simulink model "decision_stateflow"  (R2024b)
settings: Solver=ode1  StartTime=0.0  StopTime=10.0  FixedStep=0.01  RelTol=1e-3
undefined symbols (not defined in the file): U8Driver, U8DriverState, U8Ref_vel, U8RSPA, U8RSPAState
settings Model: ParamWorkspaceSource=ReferencedWorkspace  Creator=USER  LastModifiedBy=USER
settings OptimizationCC: DefaultParameterBehavior=Inlined  OptimizeBlockIOStorage=off  BufferReuse=off  ReuseModelBlockBuffer=off  GlobalBufferReuse=off  ExpressionFolding=off  EnableMemcpy=off  PassReuseOutputArgsAs=Individual arguments  LocalBlockOutputs=off  ZeroExternalMemoryAtStartup=off  ZeroInternalMemoryAtStartup=off  OptimizeDataStoreBuffers=off  BusAssignmentInplaceUpdate=off  OptimizationLevel=level0  OptimizationCustomize=off  EfficientTunableParamExpr=on
settings DebuggingCC: RTPrefix=none  ParameterTunabilityLossMsg=error  UnderSpecifiedDimensionMsg=warning
settings SFSimCC: MATLABDynamicMemAlloc=off
settings RTWCC: Description=Embedded Coder  SystemTargetFile=ert.tlc  GenCodeOnly=on  TemplateMakefile=ert_default_tmf
settings CodeAppCC: ForceParamTrailComments=on  IgnoreCustomStorageClasses=off  OperatorAnnotations=on  SimulinkDataObjDesc=on  SFDataObjDesc=on  InsertBlockDesc=on  StateflowObjectComments=on
settings ERTTargetCC: TargetLangStandard=C99 (ISO)  GenerateSampleERTMain=on  IncludeFileDelimiter=UseQuote  ERTCustomFileTemplate=example_file_process.tlc
settings ConfigComp: CovEnable=on  CovScope=Subsystem  RecordCoverage=on  CovPath=decision/StateAll

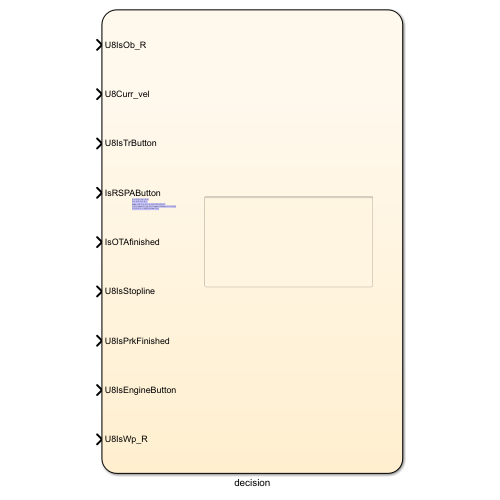
[thumbnail: Simulink's stored preview of the top-level diagram]
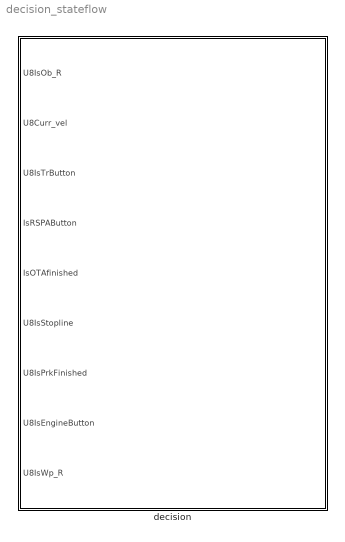
== system decision_stateflow ==
  decision : Stateflow chart  TreatAsAtomicUnit=on

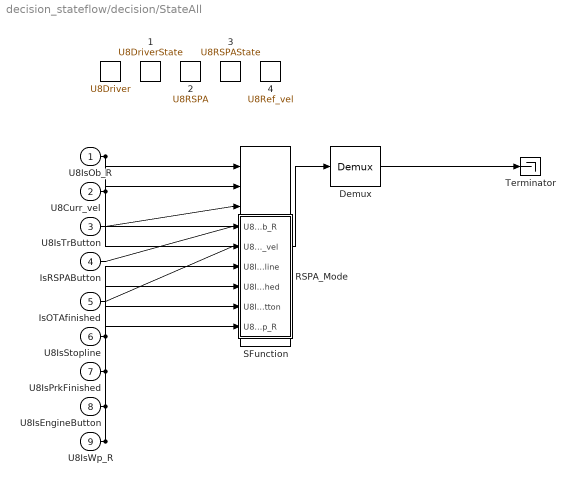
== system decision_stateflow/decision/StateAll ==
  U8IsOb_R : Inport
  U8Curr_vel : Inport  Port=2
  U8IsTrButton : Inport  Port=3
  IsRSPAButton : Inport  Port=4
  IsOTAfinished : Inport  Port=5
  U8IsStopline : Inport  Port=6
  U8IsPrkFinished : Inport  Port=7
  U8IsEngineButton : Inport  Port=8
  U8IsWp_R : Inport  Port=9
  " " : DataStoreMemory  DataStoreName=U8Driver  ShowAdditionalParam=off  OutDataTypeStr=uint8  Dimensions=[1]
  " 1" : DataStoreMemory  DataStoreName=U8DriverState  ShowAdditionalParam=off  OutDataTypeStr=uint8  Dimensions=[1]
  " 2" : DataStoreMemory  DataStoreName=U8RSPA  ShowAdditionalParam=off  OutDataTypeStr=uint8  Dimensions=[1]
  " 3" : DataStoreMemory  DataStoreName=U8RSPAState  ShowAdditionalParam=off  OutDataTypeStr=uint8  Dimensions=[1]
  " 4" : DataStoreMemory  DataStoreName=U8Ref_vel  ShowAdditionalParam=off  OutDataTypeStr=double  Dimensions=[1]
  " Demux " : Demux  Outputs=1
  " SFunction " : S-Function  Tag=Stateflow S-Function 1  FunctionName=sf_sfun  PortCounts=[9 1]  SFunctionDeploymentMode=off  EnableBusSupport=on
  " Terminator " : Terminator
  RSPA_Mode : Stateflow chart  TreatAsAtomicUnit=on  DSMNames=U8Driver,U8DriverState,U8RSPA,U8RSPAState,U8Ref_vel  DSMValues=U8Driver,U8DriverState,U8RSPA,U8RSPAState,U8Ref_vel
      settings: CopyFcn=set_param(gcbh, 'DSMNames', '', 'DSMValues', '', 'CopyFcn', '')
  wires:
  U8IsOb_R/1 -> " SFunction "/1, RSPA_Mode/1(U8IsOb_R)
  U8Curr_vel/1 -> " SFunction "/2, RSPA_Mode/2(U8Curr_vel)
  U8IsTrButton/1 -> " SFunction "/3
  IsRSPAButton/1 -> " SFunction "/4
  IsOTAfinished/1 -> " SFunction "/5
  U8IsStopline/1 -> " SFunction "/6, RSPA_Mode/3(U8IsStopline)
  U8IsPrkFinished/1 -> " SFunction "/7, RSPA_Mode/4(U8IsPrkFinished)
  U8IsEngineButton/1 -> " SFunction "/8, RSPA_Mode/5(U8IsEngineButton)
  U8IsWp_R/1 -> " SFunction "/9, RSPA_Mode/6(U8IsWp_R)
  " Demux "/1 -> " Terminator "/1
  " SFunction "/1 -> " Demux "/1

== stateflow chart decision_stateflow/decision/StateAll ==
  state SAFE_FCA
    en:
    note: 주 행중 전방 충돌방지 보조 작동,
        | 전방 초음파센서만,,
    state FCA_EMERGENCY
      en:
      U8FCAState=E;
      U8Ref_vel=0;
    state FCA_EXIT
      en:
      U8FCAState=initState;
    state FCA_DECEL
      en:
      U8FCAState=D;
      U8Ref_vel=U8Ref_vel-DTTC*(1/gainK)
    FCA_EMERGENCY -> FCA_EXIT : [U8Ref_vel == 0 ]
    FCA_DECEL -> FCA_EXIT : [U8Obs_dis >= 100 ]
  state DRIVER_Mode
    en:
    U8Driver=ModeOn;
    U8RSPA=ModeOff;
    state DRIVER_R
      en:
      U8DriverState=R;
      U8Ref_vel=DInputVR;
    state DRIVER_P
      en:
      U8DriverState=P;
      U8Ref_vel=initVel;
    note: 시동 OFF
    state DRIVER_D
      en:
      U8DriverState=D;
      U8Ref_vel=DInputVD;
    (default) -> DRIVER_P
    (junction 38) -> DRIVER_P : [U8Curr_vel==0]
    DRIVER_R -> (junction 38) [order 3] : [U8IsTrButton==0] {U8Ref_vel=0;}
    DRIVER_P -> DRIVER_D [order 1] : [U8IsTrButton==1 &&...
        |  U8Curr_vel==0]
    (junction 39) -> DRIVER_P : [U8Curr_vel==0]
    (junction 40) -> DRIVER_R : [U8Curr_vel==0]
    DRIVER_R -> (junction 41) [order 4] : [U8IsTrButton==1]
        | {U8Ref_vel=0;}
    DRIVER_R -> (junction 42) [order 5] : [IsRSPAButton==1 && IsOTAfinished ==1]
        | {U8Ref_vel=0;}
    DRIVER_D -> (junction 39) [order 1] : [U8IsTrButton==0]
        | {U8Refv=0;}
    DRIVER_D -> (junction 40) [order 2] : [U8IsTrButton==2] {U8Refv=0;}
    (junction 41) -> DRIVER_D : [U8Curr_vel==0]
    DRIVER_D -> (junction 42) [order 3] : [IsRSPAButton==1 && IsOTAfinished ==1]
        | {U8Ref_vel=0;}
  state INIT_Mode
    en:
    U8Driver=ModeOff;
    U8RSPA=ModeOff;
    U8Engine=ModeOff;
    U8DriverState=initState;
    U8RSPAState=initState;
    U8FCAState=initState;
  note: 시동 ON
  state RSPA_Mode
  state SAFE_RCA
    en:
    note: 주차중 충돌방지 보조 작동,
        | 후방 초음파센서만,,
    state RCA_EMERGENCY
      en:
      U8RCAState=E;
      U8Ref_vel=0;
    state RCA_EXIT
      en:
      U8RCAState=initState;
    state RCA_DECEL
      en:
      U8RCAState=D;
      U8Ref_vel=U8Ref_vel-DTTC*(1/gainK)
    RCA_EMERGENCY -> RCA_EXIT : [U8Ref_vel == 0 ]
    RCA_DECEL -> RCA_EXIT : [U8Obs_dis >= 100 ]
  (junction 130) -> (junction 131)
  (junction 151) -> (junction 130)
  (junction 131) -> DRIVER_R
  (default) -> INIT_Mode
  DRIVER_R -> (junction 147) [order 2] : [DTTC_R <= 1]
  (junction 147) -> (junction 148)
  (junction 108) -> FCA_EMERGENCY
  (junction 103) -> (junction 108)
  DRIVER_R -> (junction 134) [order 1] : [DTTC_R>1 && DTTC_R <=3]
  DRIVER_P -> (junction 27) [order 2] : [U8IsEngineButton==0]
  (junction 134) -> (junction 145)
  INIT_Mode -> (junction 26) : [U8IsEngineButton==1]
  (junction 26) -> DRIVER_Mode : {U8Engine=ModeOn;}
  (junction 27) -> INIT_Mode : {U8Engine=ModeOff;}
  (junction 28) -> (junction 27)
  FCA_EXIT -> (junction 124) : [U8DriverState==D]
  DRIVER_D -> (junction 103) [order 4] : [DTTC_D <= 1]
  (junction 42) -> RSPA_Mode : [U8Curr_vel==0]
  DRIVER_D -> (junction 111) [order 5] : [DTTC_D>1 && DTTC_D <=3]
  (junction 111) -> FCA_DECEL
  (junction 127) -> DRIVER_D
  (junction 124) -> (junction 127)
  (junction 148) -> RCA_EMERGENCY
  RCA_EXIT -> (junction 151) [order 1] : [U8DriverState==R]
  RCA_EXIT -> ? [order 1] : [U8DriverState==D]
  (junction 145) -> RCA_DECEL
  87 -> (junction 28)
  data: U8IsOb_R input uint8 size=1; initState constant uint8; U8Curr_vel input double size=1; U8IsTrButton input uint8; IsRSPAButton input uint8 size=1; IsOTAfinished input uint8 size=1; U8IsStopline input uint8 size=1; U8IsPrkFinished input uint8 size=1; U8IsEngineButton input uint8 size=1; ModeOff constant uint8 =0; ModeOn constant uint8 =1; U8Refv local double size=1; U8DriverState local uint8 size=1; U8Driver local uint8 size=1; R constant uint8 =2; P constant uint8 =1; D constant uint8 =0; U8Engine local uint8 size=1; U8RSPAState local uint8 size=1; U8RSPA local uint8 size=1; DInputVR constant double =-0.1; DInputVD constant double =0.1; U8IsWp_R input uint8 size=1; U8Ref_vel local double size=1; initVel constant double size=1 =0

== stateflow chart decision_stateflow/decision/StateAll/RSPA_Mode ==
  state RSPA_Mode
    en:
    U8Driver=ModeOff;
    U8RSPA=ModeOn;
    U8DriverState=initState;
    U8RSPAState=initState;
    note: 후진기어로 변경,
    state RSPA_R
      en:
      U8RSPAState=R;
      U8Ref_vel=DInputVR;
      DSteeringinput 23->0 점점 감소
    state RSPA_D
      en:
      U8RSPAState=D;
      U8Ref_vel=DInputVD;;
    state RSPA_LANE_D
      en:
      U8RSPAState=DA;
      U8Ref_vel=DInputVD;;
    note: 빈주차칸 찾으면 왼쪽 조향으로 약간 전진
    state RSPA_LANE_R
      en:
      U8RSPAState=RA;
      U8Ref_vel=DInputVR;
    state RSPA_IS_SLOT
      en:
      U8RSPAState=S;
      U8Ref_vel=DInputVD;
    note: 1. 후방에 장애물 감지시 출차
        | 2. Local wp 추종 끝났는데 주차각이 이상하면 전진-후진 삐까삐까
    note: 정지선이수평임을 감지하고 Local WP 추종이 끝났으면 Parking 완료
    state RSPA_P
      en:
      U8RSPAState=P;
    RSPA_D -> RSPA_R : [DMoveDis==0.5]
    (junction 50) -> RSPA_D : [U8Curr_vel==0] {DSteeringinput=20;}
    RSPA_R -> (junction 22) : [U8IsWp_R==1]  {U8Ref_vel=0;}
    (junction 63) -> RSPA_LANE_D [order 1]
    (junction 63) -> (junction 24) [order 2] : [U8IsStopline==1 &&...
        |  U8IsPrkFinished==1]
        | {U8Ref_vel=0;}
    (junction 22) -> RSPA_LANE_R : [U8Curr_vel==0]
    RSPA_IS_SLOT -> (junction 50) : [U8Isparkinngslot==1]{U8Ref_vel=0;}
    (junction 23) -> RSPA_LANE_D : [U8Curr_vel==0]
    RSPA_LANE_D -> (junction 56)
    (junction 56) -> RSPA_LANE_R
    (default) -> RSPA_IS_SLOT
    RSPA_LANE_R -> (junction 23) [order 2] : [U8IsOb_R==1 ||...
        |  (U8IsPrkFinished==1 && U8IsStopline==0) ]
        | {U8Ref_vel=0;}
    RSPA_LANE_R -> (junction 26) [order 1] : [U8IsStopline==1 &&...
        |  U8IsPrkFinished==1]
        | {U8Ref_vel=0;}
    (junction 24) -> (junction 25) : [U8Curr_vel==0]
    (junction 26) -> (junction 25) : [U8Curr_vel==0]
    (junction 25) -> RSPA_P
  RSPA_P -> 27 : [U8IsEngineButton==0]
  data: U8IsOb_R input uint8 size=1; initState constant uint8; U8Curr_vel input double size=1; U8IsStopline input uint8 size=1; U8IsPrkFinished input uint8 size=1; U8IsEngineButton input uint8 size=1; ModeOff constant uint8 =0; ModeOn constant uint8 =1; U8DriverState data_store_memory size=1; U8Driver data_store_memory size=1; R constant uint8 =2; P constant uint8 =1; D constant uint8 =0; U8RSPAState data_store_memory size=1; U8RSPA data_store_memory size=1; DInputVR constant double =-0.1; DInputVD constant double =0.1; U8IsWp_R input uint8 size=1; U8Ref_vel data_store_memory size=1

== stateflow chart decision_stateflow/decision ==
  state StateAll
  note: P 는 차량 속도 -0.15
      | D는 차량 속도 0.1
      | State 안에 있는 변수는 차량 제어 변수임.
      | 판단은 50ms 주기로, 제어 input 은 100ms 주기로 진행
      | 판단로직은 스케쥴링 50ms 으로,,
  data: U8IsOb_R input uint8 size=1; initState constant uint8; U8Curr_vel input double size=1; U8IsTrButton input uint8; IsRSPAButton input uint8 size=1; IsOTAfinished input uint8 size=1; U8IsStopline input uint8 size=1; U8IsPrkFinished input uint8 size=1; U8IsEngineButton input uint8 size=1; ModeOff constant uint8 =0; ModeOn constant uint8 =1; U8Refv local double size=1; U8DriverState local uint8 size=1; U8Driver local uint8 size=1; R constant uint8 =2; P constant uint8 =1; D constant uint8 =0; U8Engine local uint8 size=1; U8RSPAState local uint8 size=1; U8RSPA local uint8 size=1; DInputVR constant double =-0.1; DInputVD constant double =0.1; U8IsWp_R input uint8 size=1; U8Ref_vel local double size=1
